simulink model "SafetyChecks"  (R2020b)
settings: Solver=FixedStepDiscrete  StartTime=0.0  StopTime=10.0  FixedStep=4*Ts  RelTol=1e-3
values from neighbouring files (symbols this model uses):
  MaximumCurrentBeforeReaction = 19.0    [SafetyChecks.sldd]
libraries: simulink x3
settings Model: DataDictionary=SafetyChecks.sldd  Creator=unix  LastModifiedBy=nikotosi
settings OptimizationCC: DefaultParameterBehavior=Inlined  EnhancedBackFolding=on  PassReuseOutputArgsAs=Individual arguments  ZeroExternalMemoryAtStartup=off  ZeroInternalMemoryAtStartup=off  OptimizeBlockOrder=speed  DifferentSizesBufferReuse=on  OptimizationCustomize=off  EfficientTunableParamExpr=on
settings DebuggingCC: ParameterTunabilityLossMsg=error
settings SFSimCC: MATLABDynamicMemAlloc=off
settings RTWCC: Description=Embedded Coder  SystemTargetFile=ert.tlc  TemplateMakefile=ert_default_tmf
settings CodeAppCC: ForceParamTrailComments=on  IgnoreCustomStorageClasses=off  OperatorAnnotations=on  SimulinkDataObjDesc=on  SFDataObjDesc=on  InsertBlockDesc=on
settings ERTTargetCC: TargetLangStandard=C99 (ISO)  CodeReplacementLibrary=GNU C99 extensions  GenerateSampleERTMain=on  ArrayLayout=Row-major  InlinedParameterPlacement=NonHierarchical  ERTCustomFileTemplate=example_file_process.tlc

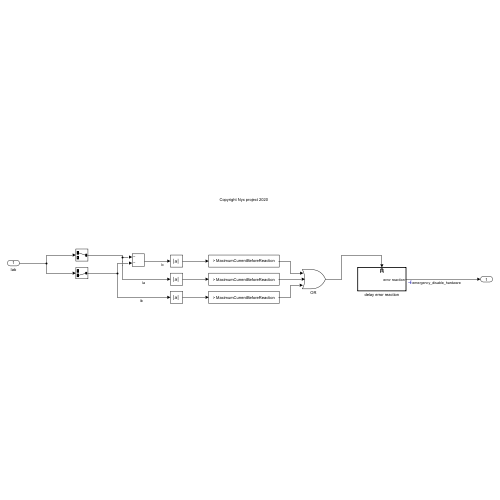
[thumbnail: Simulink's stored preview of the top-level diagram]
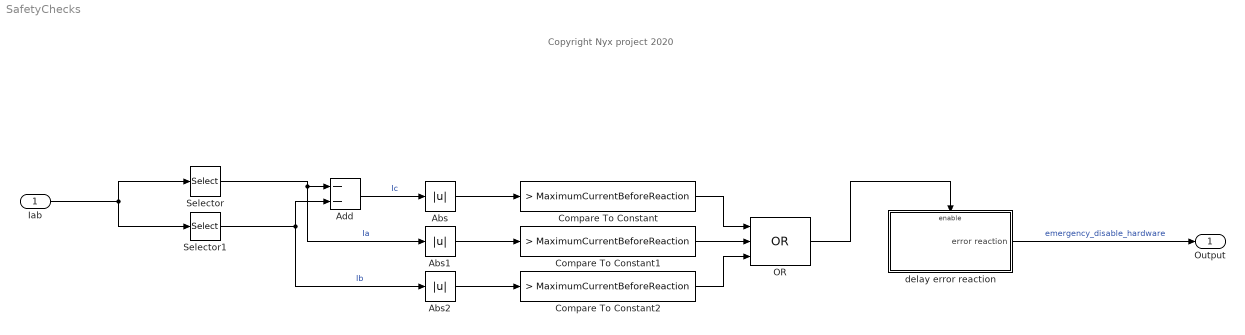
== system SafetyChecks ==
  note: Copyright Nyx project 2020
  Iab : Inport  OutDataTypeStr=single
  Abs : Abs
  Abs1 : Abs
  Abs2 : Abs
  Add : Sum  Inputs=--  RndMeth=Simplest
  Compare To Constant : simulink/Logic and Bit Operations/Compare To Constant  relop=>  const=MaximumCurrentBeforeReaction  OutDataTypeStr=boolean
  Compare To Constant1 : simulink/Logic and Bit Operations/Compare To Constant  relop=>  const=MaximumCurrentBeforeReaction  OutDataTypeStr=boolean
  Compare To Constant2 : simulink/Logic and Bit Operations/Compare To Constant  relop=>  const=MaximumCurrentBeforeReaction  OutDataTypeStr=boolean
  OR : Logic  Operator=OR  Inputs=3  IconShape=distinctive  AllPortsSameDT=off  OutDataTypeStr=boolean
  Selector : Selector  InputPortWidth=2  IndexOptions=Index vector (dialog)  Indices=[1]  OutputSizes=1
  Selector1 : Selector  InputPortWidth=2  IndexOptions=Index vector (dialog)  Indices=[2]  OutputSizes=1
  delay error reaction : Subsystem  TreatAsAtomicUnit=on
  Output : Outport
  wires:
  Iab/1 -> Selector1/1, Selector/1
  Selector/1 -> Abs1/1, Add/1  "Ia"
  Selector1/1 -> Add/2, Abs2/1  "Ib"
  Add/1 -> Abs/1  "Ic"
  Abs2/1 -> Compare To Constant2/1
  Abs1/1 -> Compare To Constant1/1
  Abs/1 -> Compare To Constant/1
  Compare To Constant1/1 -> OR/2
  Compare To Constant/1 -> OR/1
  Compare To Constant2/1 -> OR/3
  delay error reaction/1(error reaction) -> Output/1  "emergency_disable_hardware"
  OR/1 -> delay error reaction/Enable

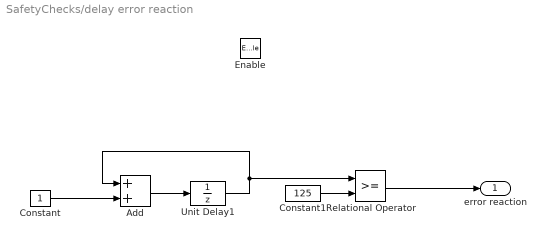
== system SafetyChecks/delay error reaction ==
  Enable : EnablePort  StatesWhenEnabling=reset
  Add : Sum  OutDataTypeStr=uint16
  Constant : Constant  OutDataTypeStr=uint8
  Constant1 : Constant  Value=125  OutDataTypeStr=uint16
  Relational Operator : RelationalOperator  OutDataTypeStr=boolean  RndMeth=Simplest
  Unit Delay1 : UnitDelay  SampleTime=-1  HasFrameUpgradeWarning=on
  error reaction : Outport  OutputWhenDisabled=reset  InitialOutput=0
      settings: AttributesFormatString=%<InitialOutput>
  wires:
  Add/1 -> Unit Delay1/1
  Unit Delay1/1 -> Relational Operator/1, Add/1
  Constant/1 -> Add/2
  Constant1/1 -> Relational Operator/2
  Relational Operator/1 -> error reaction/1
